simulink model "Lab9"  (R2022a)
settings: Solver=FixedStepAuto  StartTime=0.0  StopTime=20  FixedStep=Ts  MinStep=1e-3  RelTol=1e-3
undefined symbols (not defined in the file): kP, kPI, kPID, poles, Td, Ti1, Ti2
settings Model: Creator=ishaan  LastModifiedBy=ishaan

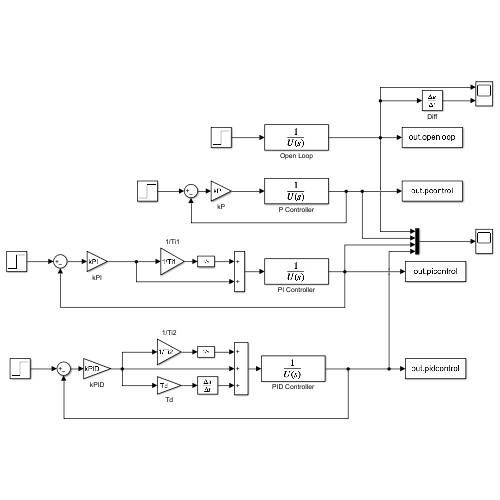
[thumbnail: Simulink's stored preview of the top-level diagram]
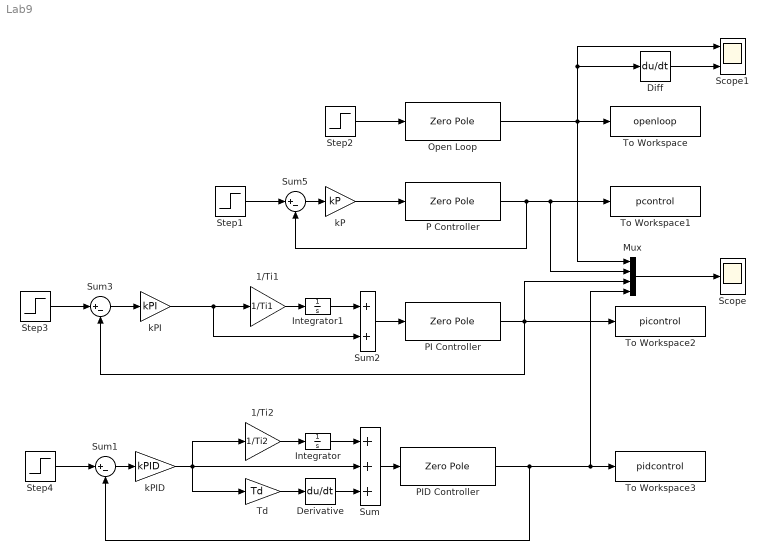
== system Lab9 ==
  1/Ti1 : Gain  Gain=1/Ti1
  1/Ti2 : Gain  Gain=1/Ti2
  Derivative : Derivative
  Diff : Derivative
  Integrator : Integrator
  Integrator1 : Integrator
  Mux : Mux
  Open Loop : ZeroPole  Zeros=[]  Poles=poles
  P Controller : ZeroPole  Zeros=[]  Poles=poles
  PI Controller : ZeroPole  Zeros=[]  Poles=poles
  PID Controller : ZeroPole  Zeros=[]  Poles=poles
  Scope : Scope
  Scope1 : Scope  NumInputPorts=2
  Step{1..4} (4 alike) : Step  Time=0  SampleTime=0
  Sum : Sum  Inputs=+++
  Sum1 : Sum  Inputs=|+-
  Sum2 : Sum
  Sum3 : Sum  Inputs=|+-
  Sum5 : Sum  Inputs=|+-
  Td : Gain  Gain=Td
  To Workspace : ToWorkspace  VariableName=openloop  SaveFormat=Structure With Time  SampleTime=-1
  To Workspace1 : ToWorkspace  VariableName=pcontrol  SaveFormat=Structure With Time  SampleTime=-1
  To Workspace2 : ToWorkspace  VariableName=picontrol  SaveFormat=Structure With Time  SampleTime=-1
  To Workspace3 : ToWorkspace  VariableName=pidcontrol  SaveFormat=Structure With Time  SampleTime=-1
  kP : Gain  Gain=kP
  kPI : Gain  Gain=kPI
  kPID : Gain  Gain=kPID
  wires:
  PID Controller/1 -> To Workspace3/1, Mux/4, Sum1/2
  Sum/1 -> PID Controller/1
  kPID/1 -> Td/1, Sum/2, 1/Ti2/1
  Derivative/1 -> Sum/3
  Integrator/1 -> Sum/1
  Sum1/1 -> kPID/1
  1/Ti2/1 -> Integrator/1
  Td/1 -> Derivative/1
  Step2/1 -> Open Loop/1
  1/Ti1/1 -> Integrator1/1
  Sum3/1 -> kPI/1
  Integrator1/1 -> Sum2/1
  kPI/1 -> Sum2/2, 1/Ti1/1
  Sum2/1 -> PI Controller/1
  PI Controller/1 -> To Workspace2/1, Mux/3, Sum3/2
  P Controller/1 -> Sum5/2, To Workspace1/1, Mux/2
  Sum5/1 -> kP/1
  kP/1 -> P Controller/1
  Step1/1 -> Sum5/1
  Step3/1 -> Sum3/1
  Step4/1 -> Sum1/1
  Open Loop/1 -> To Workspace/1, Diff/1, Scope1/1, Mux/1
  Mux/1 -> Scope/1
  Diff/1 -> Scope1/2
